simulink model "nonlinear_obs_primaldual_2019b"  (R2019b)
settings: Solver=VariableStepAuto  StartTime=0.0  StopTime=500  RelTol=1e-3
values from neighbouring files (symbols this model uses):
  alpha = Vmax/umax    (= 7.33333333333)    [PrimalDualVariableHorizon.m]    (also in QuadTankDriver.m; Simulate_QT_Simulink_MPC_LECO.m)
  Ao1 = pi * Do1^2 / 4    (= 0.17813934812)    [Simulate_QT_Simulink_MPC_LECO.m]
  Ao2 = pi * Do2^2 / 4    (= 0.17813934812)    [Simulate_QT_Simulink_MPC_LECO.m]
  Ao3 = pi * Do3^2 / 4    (= 0.17813934812)    [Simulate_QT_Simulink_MPC_LECO.m]
  Ao4 = pi * Do4^2 / 4    (= 0.17813934812)    [Simulate_QT_Simulink_MPC_LECO.m]
  At1 = pi * Dt1^2 / 4    (= 15.5179165474)    [Simulate_QT_Simulink_MPC_LECO.m]
  At2 = pi * Dt2^2 / 4    (= 15.5179165474)    [Simulate_QT_Simulink_MPC_LECO.m]
  At3 = pi * Dt3^2 / 4    (= 15.5179165474)    [Simulate_QT_Simulink_MPC_LECO.m]
  At4 = pi * Dt4^2 / 4    (= 15.5179165474)    [Simulate_QT_Simulink_MPC_LECO.m]
  g = 981    [Simulate_QT_Simulink_MPC.m]    (also in Simulate_QT_Simulink_MPC_LECO.m; Simulate_QuadTank_MPC.m)
  gamma1 = Ai1/(Ai1+Ai4)    (= 0.64)    [Simulate_QT_Simulink_MPC_LECO.m]
  gamma2 = Ai2/(Ai2+Ai3)    (= 0.64)    [Simulate_QT_Simulink_MPC_LECO.m]
  Kp = 3.3    [Simulate_QT_Simulink_MPC_LECO.m]
  Ld = Ltemp(n+1:end,:)    [PrimalDual_setup.m]
  Lx = Ltemp(1:n,:)    [PrimalDual_setup.m]
  m = size(Bc,2)    [MPCTool_setup.m]    (also in PrimalDualVariableHorizon.m; PrimalDual_setup.m; QuadTankDriver.m)
  Np = Np3    [PrimalDualVariableHorizon.m]    (also in QuadTankDriver.m = 5)
  umax = 3    [PrimalDualVariableHorizon.m]    (also in QuadTankDriver.m; Simulate_QT_Simulink_MPC_LECO.m)
undefined symbols (not defined in the file or in its folder): Ac, Bc, Cc, F1, F2, F3, H, L10, L20, Vp10, Vp20
settings Model: Creator=frankiemoran  LastModifiedBy=adegbega

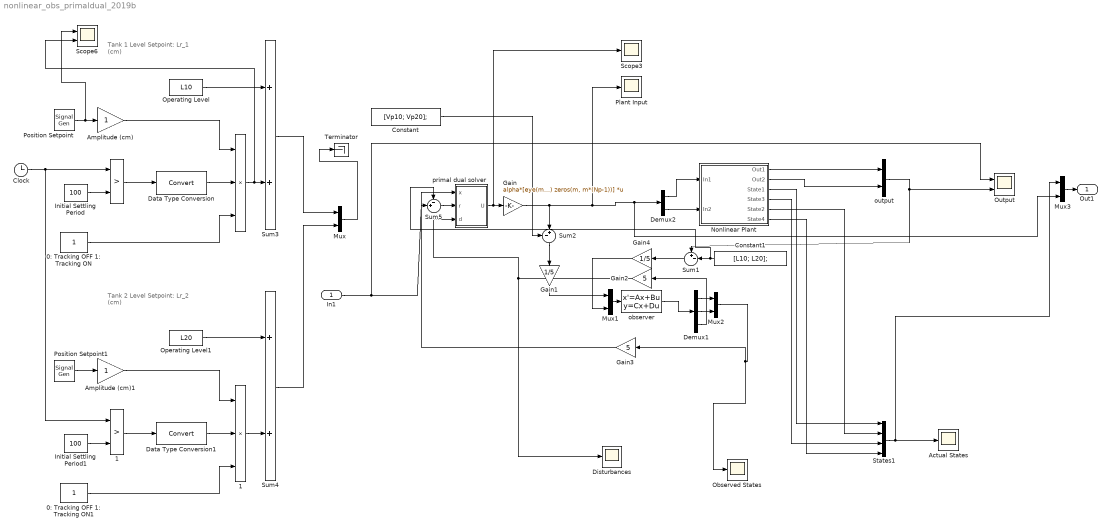
== system nonlinear_obs_primaldual_2019b ==
  note: Tank 2 Level Setpoint:
      | Lr_2 (cm)
  note: Tank 1 Level Setpoint:
      | Lr_1 (cm)
  In1 : Inport  PortDimensions=2
  "   " : Product  Inputs=3  SaturateOnIntegerOverflow=on  RndMeth=Zero  InputSameDT=on  OutDataTypeStr=Inherit: Same as first input
  "    " : RelationalOperator  Operator=>  RndMeth=Nearest  InputSameDT=on
  "    1" : RelationalOperator  Operator=>  RndMeth=Nearest  InputSameDT=on
  "   1" : Product  Inputs=3  SaturateOnIntegerOverflow=on  RndMeth=Zero  InputSameDT=on  OutDataTypeStr=Inherit: Same as first input
  0: Tracking OFF 1: Tracking ON : Constant
  0: Tracking OFF 1: Tracking ON1 : Constant
  Actual States : Scope
  Amplitude (cm) : Gain  SaturateOnIntegerOverflow=on  OutDataTypeStr=Inherit: Same as input  ParamDataTypeStr=Inherit: Same as input
  Amplitude (cm)1 : Gain  SaturateOnIntegerOverflow=on  OutDataTypeStr=Inherit: Same as input  ParamDataTypeStr=Inherit: Same as input
  Clock : Clock
  Constant : Constant  Value=[Vp10; Vp20];
  Constant1 : Constant  Value=[L10; L20];
  Data Type Conversion : DataTypeConversion
  Data Type Conversion1 : DataTypeConversion
  Demux1 : Demux  Outputs=3
  Demux2 : Demux  Outputs=2
  Disturbances : Scope
  Gain : Gain  Gain=alpha*[eye(m) zeros(m, m*(Np-1))]  Multiplication=Matrix(K*u)
  Gain1 : Gain  Gain=1/5
  Gain2 : Gain  Gain=5
  Gain3 : Gain  Gain=5
  Gain4 : Gain  Gain=1/5
  Initial Settling Period : Constant  Value=100
  Initial Settling Period1 : Constant  Value=100
  Mux{,1..3} (4 alike) : Mux  Inputs=2
  Nonlinear Plant : Subsystem
  Observed States : Scope
  Operating Level : Constant  Value=L10
  Operating Level1 : Constant  Value=L20
  Output : Scope  NumInputPorts=2
  Plant Input : Scope
  Position Setpoint : SignalGenerator  WaveForm=square  Frequency=0.018/4
  Position Setpoint1 : SignalGenerator  WaveForm=square  Frequency=0.018/4
  Scope3 : Scope
  Scope6 : Scope  NumInputPorts=2
  States1 : Mux
  Sum1 : Sum  Inputs=+-|
  Sum2 : Sum  Inputs=-+|
  Sum3 : Sum  SaturateOnIntegerOverflow=on  InputSameDT=on  OutDataTypeStr=Inherit: Same as first input
  Sum4 : Sum  SaturateOnIntegerOverflow=on  InputSameDT=on  OutDataTypeStr=Inherit: Same as first input
  Sum5 : Sum  Inputs=-+|
  Terminator : Terminator
  observer : StateSpace  A=[Ac-Lx*Cc -Lx; -Ld*Cc -Ld];  B=[Bc +Lx; zeros(2) +Ld];  C=eye(6)  D=zeros(6, 4);  InitialCondition=0
  output : Mux  Inputs=2
  "primal dual solver " : Subsystem
  Out1 : Outport
  wires:
  observer/1 -> Demux1/1
  Amplitude (cm)1/1 -> "   1"/1
  Mux1/1 -> observer/1
  0: Tracking OFF 1: Tracking ON1/1 -> "   1"/3
  Position Setpoint/1 -> Scope6/1, Amplitude (cm)/1
  Amplitude (cm)/1 -> "   "/1
  Sum1/1 -> Gain4/1
  Position Setpoint1/1 -> Amplitude (cm)1/1
  Data Type Conversion1/1 -> "   1"/2
  0: Tracking OFF 1: Tracking ON/1 -> "   "/3
  Initial Settling Period/1 -> "    "/2
  Clock/1 -> "    "/1, "    1"/1
  Operating Level/1 -> Sum3/1
  Initial Settling Period1/1 -> "    1"/2
  Data Type Conversion/1 -> "   "/2
  "    1"/1 -> Data Type Conversion1/1
  Operating Level1/1 -> Sum4/1
  "    "/1 -> Data Type Conversion/1
  Sum3/1 -> Mux/1
  Sum4/1 -> Mux/2
  Demux1/1 -> Mux2/1
  Demux1/2 -> Mux2/2
  Mux2/1 -> Gain3/1, Observed States/1
  Demux1/3 -> Gain2/1
  Demux2/1 -> Nonlinear Plant/1(In1)
  Demux2/2 -> Nonlinear Plant/2(In2)
  Nonlinear Plant/3(State1) -> States1/1
  Nonlinear Plant/6(State4) -> States1/4
  States1/1 -> Mux3/1, Actual States/1
  Nonlinear Plant/2(Out2) -> output/2
  Nonlinear Plant/1(Out1) -> output/1
  output/1 -> Sum1/1, Output/2
  "   "/1 -> Scope6/2, Sum3/2
  "   1"/1 -> Sum4/2
  "primal dual solver "/1(U) -> Scope3/1, Gain/1
  Gain/1 -> Sum2/2, Plant Input/1, Mux3/2, Demux2/1
  Sum5/1 -> "primal dual solver "/2(r)
  Sum2/1 -> Gain1/1
  Constant/1 -> Sum2/1
  Gain1/1 -> Mux1/1
  Gain3/1 -> "primal dual solver "/1(x)
  Gain2/1 -> "primal dual solver "/3("d "), Disturbances/1
  Constant1/1 -> Sum5/1, Sum1/2
  Gain4/1 -> Mux1/2
  Mux/1 -> Terminator/1
  In1/1 -> Output/1, Sum5/2
  Mux3/1 -> Out1/1
  Nonlinear Plant/5(State2) -> States1/2
  Nonlinear Plant/4(State3) -> States1/3

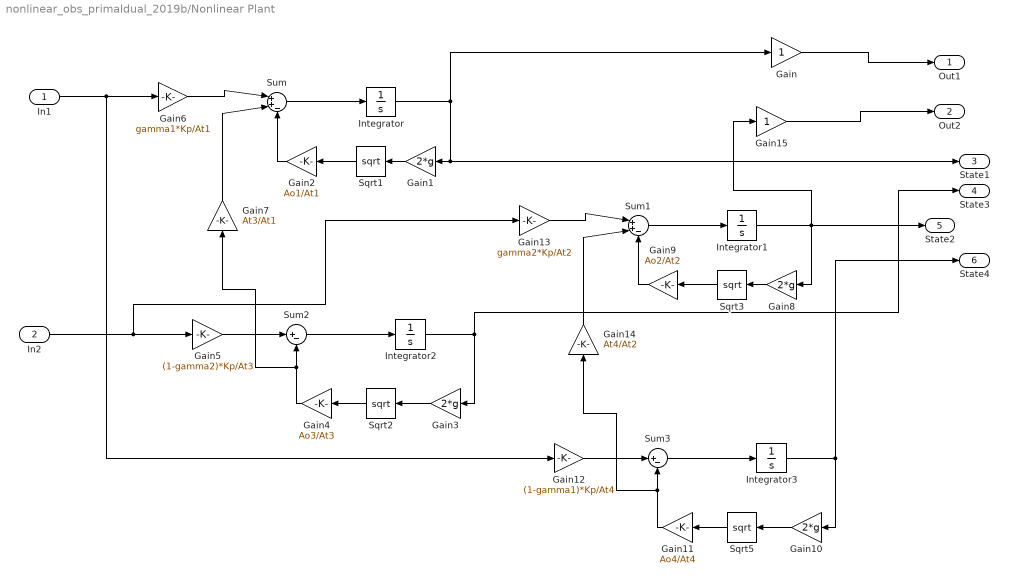
== system nonlinear_obs_primaldual_2019b/Nonlinear Plant ==
  In1 : Inport
  In2 : Inport  Port=2
  Gain : Gain
  Gain{1,3,8,10} (4 alike) : Gain  Gain=2*g
  Gain11 : Gain  Gain=Ao4/At4
  Gain12 : Gain  Gain=(1-gamma1)*Kp/At4
  Gain13 : Gain  Gain=gamma2*Kp/At2
  Gain14 : Gain  Gain=At4/At2
  Gain15 : Gain
  Gain2 : Gain  Gain=Ao1/At1
  Gain4 : Gain  Gain=Ao3/At3
  Gain5 : Gain  Gain=(1-gamma2)*Kp/At3
  Gain6 : Gain  Gain=gamma1*Kp/At1
  Gain7 : Gain  Gain=At3/At1
  Gain9 : Gain  Gain=Ao2/At2
  Integrator{,1..3} (4 alike) : Integrator
  Sqrt{1..3,5} (4 alike) : Sqrt  SaturateOnIntegerOverflow=on
  Sum : Sum  Inputs=|++-
  Sum1 : Sum  Inputs=|++-
  Sum2 : Sum  Inputs=|+-
  Sum3 : Sum  Inputs=|+-
  Out1 : Outport
  Out2 : Outport  Port=2
  State1 : Outport  Port=3
  State3 : Outport  Port=4
  State2 : Outport  Port=5
  State4 : Outport  Port=6
  wires:
  Gain14/1 -> Sum1/2
  Gain/1 -> Out1/1
  In2/1 -> Gain13/1, Gain5/1
  Gain13/1 -> Sum1/1
  Gain8/1 -> Sqrt3/1
  Sqrt3/1 -> Gain9/1
  Sum1/1 -> Integrator1/1
  Gain9/1 -> Sum1/3
  Integrator3/1 -> State4/1, Gain10/1
  Integrator2/1 -> State3/1, Gain3/1
  Gain12/1 -> Sum3/1
  Gain3/1 -> Sqrt2/1
  In1/1 -> Gain12/1, Gain6/1
  Sum3/1 -> Integrator3/1
  Gain5/1 -> Sum2/1
  Gain11/1 -> Gain14/1, Sum3/2
  Integrator1/1 -> Gain15/1, State2/1, Gain8/1
  Integrator/1 -> State1/1, Gain1/1, Gain/1
  Gain2/1 -> Sum/3
  Gain15/1 -> Out2/1
  Gain4/1 -> Gain7/1, Sum2/2
  Sum2/1 -> Integrator2/1
  Sqrt1/1 -> Gain2/1
  Sum/1 -> Integrator/1
  Gain6/1 -> Sum/1
  Gain1/1 -> Sqrt1/1
  Sqrt2/1 -> Gain4/1
  Gain7/1 -> Sum/2
  Gain10/1 -> Sqrt5/1
  Sqrt5/1 -> Gain11/1

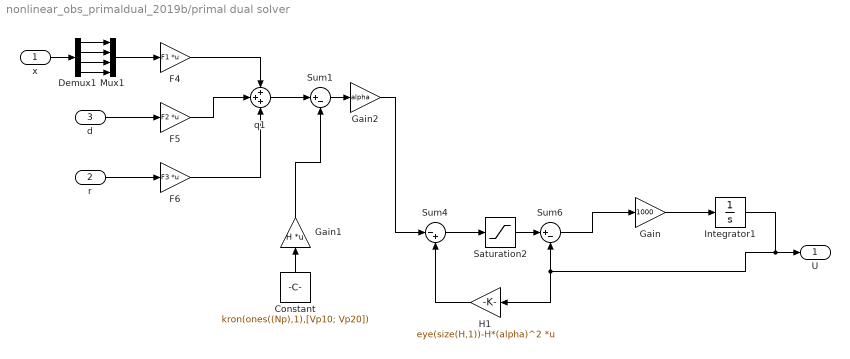
== system nonlinear_obs_primaldual_2019b/primal dual solver  ==
  x : Inport
  r : Inport  Port=2
  "d " : Inport  Port=3
  Constant : Constant  Value=kron(ones((Np),1),[Vp10; Vp20])
  Demux1 : Demux
  F4 : Gain  Gain=F1  Multiplication=Matrix(K*u)
  F5 : Gain  Gain=F2  Multiplication=Matrix(K*u)
  F6 : Gain  Gain=F3  Multiplication=Matrix(K*u)
  Gain : Gain  Gain=1000
  Gain1 : Gain  Gain=H  Multiplication=Matrix(K*u)
  Gain2 : Gain  Gain=alpha
  H1 : Gain  Gain=eye(size(H,1))-H*(alpha)^2  Multiplication=Matrix(K*u)
  Integrator1 : Integrator
  Mux1 : Mux
  Saturation2 : Saturate  UpperLimit=umax  LowerLimit=0
  Sum1 : Sum  Inputs=|+-
  Sum4 : Sum  Inputs=|-+
  Sum6 : Sum  Inputs=|+-
  q1 : Sum  Inputs=+++
  U : Outport
  wires:
  F5/1 -> q1/2
  x/1 -> Demux1/1
  Demux1/1 -> Mux1/1
  "d "/1 -> F5/1
  F6/1 -> q1/3
  r/1 -> F6/1
  Demux1/4 -> Mux1/4
  Mux1/1 -> F4/1
  Demux1/3 -> Mux1/3
  Demux1/2 -> Mux1/2
  F4/1 -> q1/1
  Saturation2/1 -> Sum6/1
  Sum6/1 -> Gain/1
  H1/1 -> Sum4/2
  Sum4/1 -> Saturation2/1
  Integrator1/1 -> H1/1, Sum6/2, U/1
  Gain/1 -> Integrator1/1
  q1/1 -> Sum1/1
  Sum1/1 -> Gain2/1
  Constant/1 -> Gain1/1
  Gain1/1 -> Sum1/2
  Gain2/1 -> Sum4/1
